simulink model "balanceCar"  (R2023b)
settings: Solver=VariableStepAuto  StartTime=0.0  StopTime=40  RelTol=1e-3
settings Model: Creator=xjtu  LastModifiedBy=xjtu

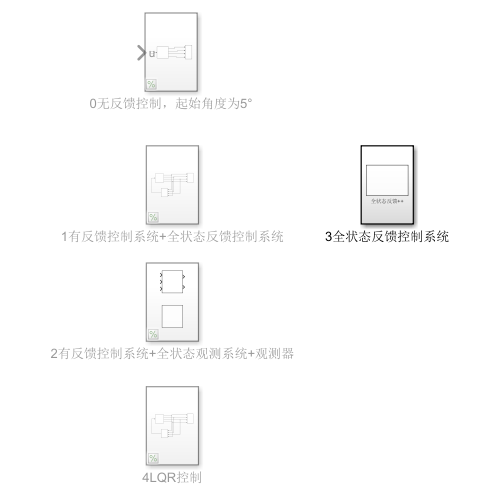
[thumbnail: Simulink's stored preview of the top-level diagram]
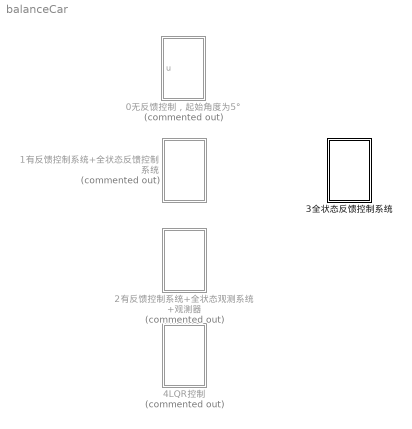
== system balanceCar ==
  0无反馈控制，起始角度为5° : Subsystem  Commented=on
  1有反馈控制系统+全状态反馈控制系统 : Subsystem  Commented=on
  2有反馈控制系统+全状态观测系统+观测器 : Subsystem  Commented=on
  3全状态反馈控制系统 : Subsystem
  4LQR控制 : Subsystem  Commented=on

== system balanceCar/0无反馈控制，起始角度为5° ==
  u : Inport
  Scope : Scope  NumInputPorts=4
  Subsystem : Subsystem
  wires:
  Subsystem/4(dot theta) -> Scope/4
  Subsystem/1(x) -> Scope/1
  u/1 -> Subsystem/1(u)
  Subsystem/2(dot x) -> Scope/2
  Subsystem/3(theta) -> Scope/3

== system balanceCar/1有反馈控制系统+全状态反馈控制系统 ==
  Scope : Scope  NumInputPorts=4
  Subsystem : Subsystem
  Subsystem1 : Subsystem
  wires:
  Subsystem1/3(theta) -> Scope/3, Subsystem/3(theta)
  Subsystem1/4(dot theta) -> Scope/4, Subsystem/4(dot theta)
  Subsystem1/2(dot x) -> Scope/2, Subsystem/2(dot x)
  Subsystem1/1(x) -> Subsystem/1(x), Scope/1
  Subsystem/1(u) -> Subsystem1/1(u)

== system balanceCar/2有反馈控制系统+全状态观测系统+观测器 ==
  全状态观测++ : Subsystem
  可以用来参考学习 : Subsystem

== system balanceCar/3全状态反馈控制系统 ==
  全状态反馈++ : Subsystem

== system balanceCar/4LQR控制 ==
  Scope : Scope  NumInputPorts=4
  Subsystem : Subsystem
  Subsystem1 : Subsystem
  wires:
  Subsystem/1(u) -> Subsystem1/1(u)
  Subsystem1/1(x) -> Scope/1, Subsystem/1(x)
  Subsystem1/2(dot x) -> Subsystem/2(dot x), Scope/2
  Subsystem1/4(dot theta) -> Subsystem/4(dot theta), Scope/4
  Subsystem1/3(theta) -> Subsystem/3(theta), Scope/3

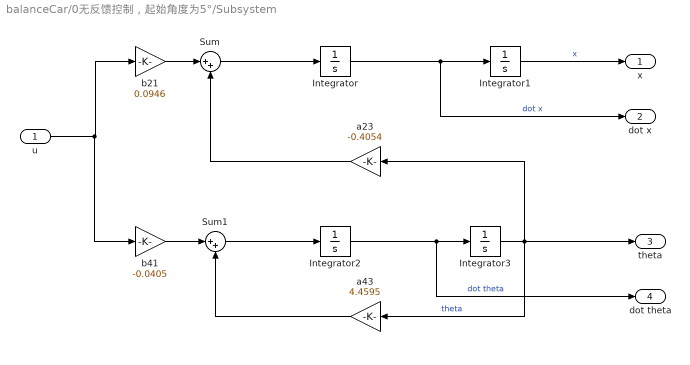
== system balanceCar/0无反馈控制，起始角度为5°/Subsystem ==
  u : Inport
  Integrator : Integrator
  Integrator1 : Integrator
  Integrator2 : Integrator
  Integrator3 : Integrator  InitialCondition=5*pi/180  UpperSaturationLimit=360  LowerSaturationLimit=-360
  Sum : Sum  Inputs=|++
  Sum1 : Sum  Inputs=|++
  a23 : Gain  Gain=-0.4054
  a43 : Gain  Gain=4.4595
  b21 : Gain  Gain=0.0946
  b41 : Gain  Gain=-0.0405
  x : Outport
  dot x : Outport  Port=2
  theta : Outport  Port=3
  dot theta : Outport  Port=4
  wires:
  Integrator2/1 -> dot theta/1, Integrator3/1  "dot theta"
  u/1 -> b41/1, b21/1
  Sum1/1 -> Integrator2/1
  Integrator1/1 -> x/1  "x"
  a23/1 -> Sum/2
  b21/1 -> Sum/1
  Integrator/1 -> dot x/1, Integrator1/1  "dot x"
  Integrator3/1 -> theta/1, a43/1, a23/1  "theta"
  b41/1 -> Sum1/1
  Sum/1 -> Integrator/1
  a43/1 -> Sum1/2

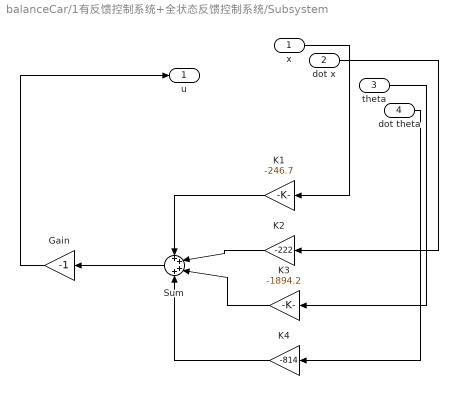
== system balanceCar/1有反馈控制系统+全状态反馈控制系统/Subsystem ==
  x : Inport
  dot x : Inport  Port=2
  theta : Inport  Port=3
  dot theta : Inport  Port=4
  Gain : Gain  Gain=-1
  K1 : Gain  Gain=-246.7
  K2 : Gain  Gain=-222
  K3 : Gain  Gain=-1894.2
  K4 : Gain  Gain=-814
  Sum : Sum  Inputs=++++
  u : Outport
  wires:
  dot theta/1 -> K4/1
  Gain/1 -> u/1
  K2/1 -> Sum/2
  Sum/1 -> Gain/1
  x/1 -> K1/1
  K1/1 -> Sum/1
  K3/1 -> Sum/3
  dot x/1 -> K2/1
  K4/1 -> Sum/4
  theta/1 -> K3/1

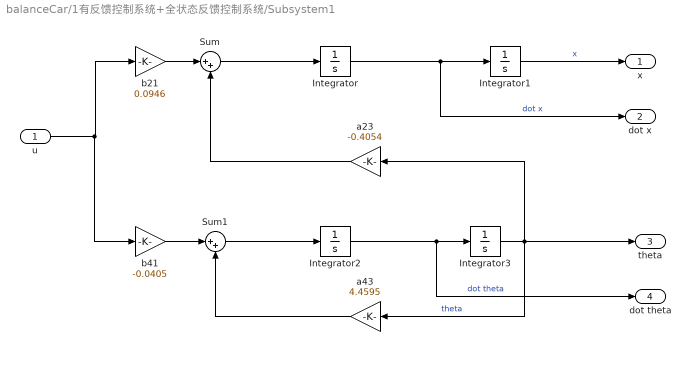
== system balanceCar/1有反馈控制系统+全状态反馈控制系统/Subsystem1 ==
  u : Inport
  Integrator : Integrator
  Integrator1 : Integrator
  Integrator2 : Integrator
  Integrator3 : Integrator  InitialCondition=5*pi/180  UpperSaturationLimit=360  LowerSaturationLimit=-360
  Sum : Sum  Inputs=|++
  Sum1 : Sum  Inputs=|++
  a23 : Gain  Gain=-0.4054
  a43 : Gain  Gain=4.4595
  b21 : Gain  Gain=0.0946
  b41 : Gain  Gain=-0.0405
  x : Outport
  dot x : Outport  Port=2
  theta : Outport  Port=3
  dot theta : Outport  Port=4
  wires:
  a43/1 -> Sum1/2
  Sum/1 -> Integrator/1
  b41/1 -> Sum1/1
  Integrator3/1 -> a23/1, a43/1, theta/1  "theta"
  Integrator/1 -> Integrator1/1, dot x/1  "dot x"
  b21/1 -> Sum/1
  a23/1 -> Sum/2
  Integrator1/1 -> x/1  "x"
  Sum1/1 -> Integrator2/1
  u/1 -> b21/1, b41/1
  Integrator2/1 -> Integrator3/1, dot theta/1  "dot theta"

== system balanceCar/2有反馈控制系统+全状态观测系统+观测器/全状态观测++ ==
  Scope : Scope  NumInputPorts=4
  Subsystem : Subsystem
  Subsystem1 : Subsystem
  Subsystem2 : Subsystem
  位移对比 : Scope  NumInputPorts=2
  角度对比 : Scope  NumInputPorts=2
  角速度对比 : Scope  NumInputPorts=2
  速度对比 : Scope  NumInputPorts=2
  wires:
  Subsystem1/2(dot x) -> Scope/2, 速度对比/1, Subsystem/2(dot x)
  Subsystem1/4(dot theta) -> Scope/4, 角速度对比/1, Subsystem/4(dot theta)
  Subsystem/1(u) -> Subsystem1/1(u)
  Subsystem1/1(x) -> Subsystem2/1(x), 位移对比/1, Scope/1, Subsystem/1(x)
  Subsystem1/3(theta) -> Subsystem2/2(theta), Scope/3, 角度对比/1, Subsystem/3(theta)
  Subsystem2/1(位移x) -> 位移对比/2
  Subsystem2/3(角度 theta) -> 角度对比/2
  Subsystem2/2(速度 dot x) -> 速度对比/2
  Subsystem2/4(角速度 dot theta) -> 角速度对比/2

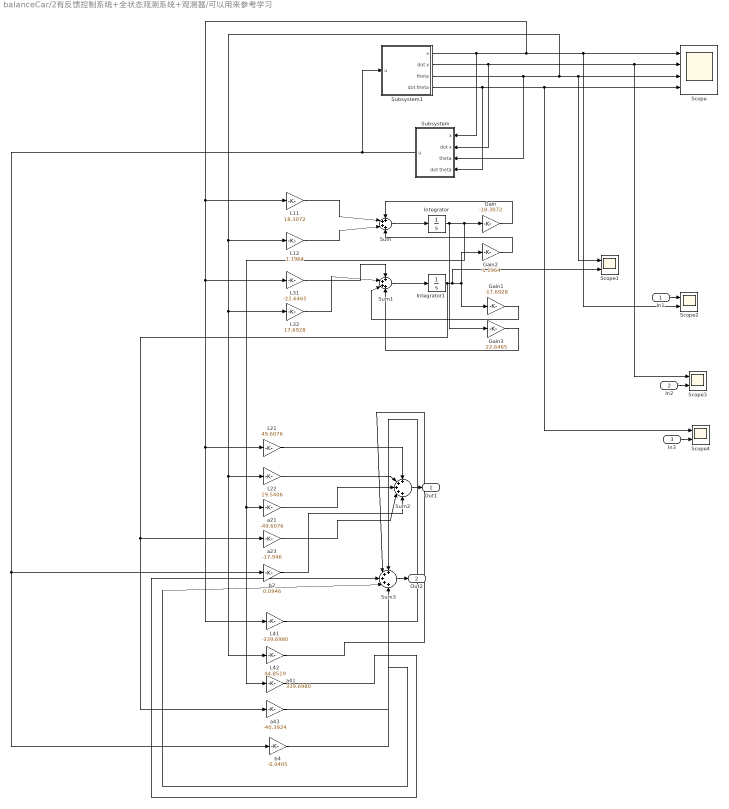
== system balanceCar/2有反馈控制系统+全状态观测系统+观测器/可以用来参考学习 ==
  In1 : Inport
  In2 : Inport  Port=2
  In3 : Inport  Port=3
  Gain : Gain  Gain=-18.3072
  Gain1 : Gain  Gain=-17.6928
  Gain2 : Gain  Gain=-1.1964
  Gain3 : Gain  Gain=22.6465
  Integrator : Integrator
  Integrator1 : Integrator  InitialCondition=pi*5/180
  L11 : Gain  Gain=18.3072
  L12 : Gain  Gain=1.1964
  L21 : Gain  Gain=49.6076
  L22 : Gain  Gain=19.5406
  L31 : Gain  Gain=-22.6465
  L32 : Gain  Gain=17.6928
  L41 : Gain  Gain=-339.6980
  L42 : Gain  Gain=44.8519
  Scope : Scope  NumInputPorts=4
  Scope{1..4} (4 alike) : Scope  NumInputPorts=2
  Subsystem : Subsystem
  Subsystem1 : Subsystem
  Sum : Sum  Inputs=++++
  Sum1 : Sum  Inputs=++++
  Sum2 : Sum  Inputs=+++++
  Sum3 : Sum  Inputs=+++++
  a21 : Gain  Gain=-49.6076
  a23 : Gain  Gain=-17.946
  a41 : Gain  Gain=339.6980
  a43 : Gain  Gain=-40.3924
  b2 : Gain  Gain=0.0946
  b4 : Gain  Gain=-0.0405
  Out1 : Outport
  Out2 : Outport  Port=2
  wires:
  L11/1 -> Sum/2
  L21/1 -> Sum2/1
  Subsystem1/3(theta) -> Subsystem/3(theta), L32/1, L22/1, L42/1, L12/1, Scope1/1, Scope/3
  Gain3/1 -> Sum1/4
  a43/1 -> Sum3/4
  Subsystem1/1(x) -> Subsystem/1(x), L31/1, L21/1, L41/1, L11/1, Scope/1, Scope2/2
  b4/1 -> Sum3/5
  Gain2/1 -> Sum/4
  a41/1 -> Sum3/3
  Integrator1/1 -> Gain2/1, Gain1/1, Scope1/2, a43/1, a23/1
  L42/1 -> Sum3/2
  L22/1 -> Sum2/2
  L32/1 -> Sum1/2
  L31/1 -> Sum1/1
  Subsystem/1(u) -> Subsystem1/1(u), b2/1, b4/1
  Subsystem1/4(dot theta) -> Subsystem/4(dot theta), Scope4/1, Scope/4
  In2/1 -> Scope3/2
  Sum/1 -> Integrator/1
  a23/1 -> Sum2/4
  Subsystem1/2(dot x) -> Subsystem/2(dot x), Scope3/1, Scope/2
  L41/1 -> Sum3/1
  L12/1 -> Sum/3
  Integrator/1 -> Gain3/1, a41/1, a21/1, Gain/1
  Sum1/1 -> Integrator1/1
  b2/1 -> Sum2/5
  a21/1 -> Sum2/3
  Gain/1 -> Sum/1
  Gain1/1 -> Sum1/3
  Sum2/1 -> Out1/1
  Sum3/1 -> Out2/1
  In1/1 -> Scope2/1
  In3/1 -> Scope4/2

== system balanceCar/3全状态反馈控制系统/全状态反馈++ ==
  Scope : Scope  NumInputPorts=4
  Subsystem : Subsystem
  Subsystem1 : Subsystem
  Subsystem2 : Subsystem
  位移对比 : Scope  NumInputPorts=2
  角度对比 : Scope  NumInputPorts=2
  角速度对比 : Scope  NumInputPorts=2
  速度对比 : Scope  NumInputPorts=2
  wires:
  Subsystem1/2(dot x) -> 速度对比/1, Scope/2, Subsystem/2(dot x)
  Subsystem2/4(角速度 dot theta) -> 角速度对比/2
  Subsystem1/3(theta) -> Subsystem/3(theta), 角度对比/1, Scope/3, Subsystem2/2(theta)
  Subsystem1/1(x) -> Subsystem/1(x), Scope/1, 位移对比/1, Subsystem2/1(x)
  Subsystem/1(u) -> Subsystem1/1(u)
  Subsystem2/1(位移x) -> 位移对比/2
  Subsystem2/3(角度 theta) -> 角度对比/2
  Subsystem2/2(速度 dot x) -> 速度对比/2
  Subsystem1/4(dot theta) -> Subsystem/4(dot theta), 角速度对比/1, Scope/4

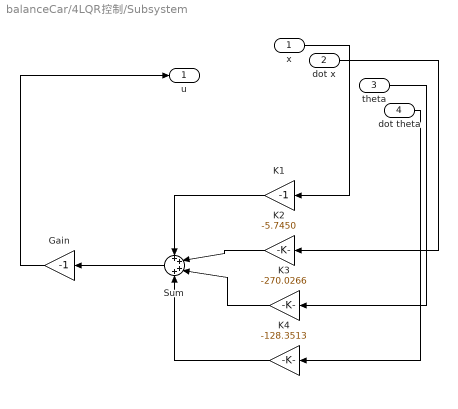
== system balanceCar/4LQR控制/Subsystem ==
  x : Inport
  dot x : Inport  Port=2
  theta : Inport  Port=3
  dot theta : Inport  Port=4
  Gain : Gain  Gain=-1
  K1 : Gain  Gain=-1
  K2 : Gain  Gain=-5.7450
  K3 : Gain  Gain=-270.0266
  K4 : Gain  Gain=-128.3513
  Sum : Sum  Inputs=++++
  u : Outport
  wires:
  theta/1 -> K3/1
  K4/1 -> Sum/4
  dot x/1 -> K2/1
  K3/1 -> Sum/3
  K1/1 -> Sum/1
  x/1 -> K1/1
  Sum/1 -> Gain/1
  K2/1 -> Sum/2
  Gain/1 -> u/1
  dot theta/1 -> K4/1

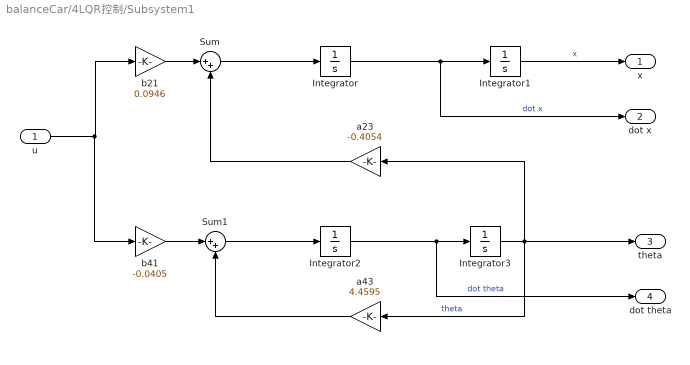
== system balanceCar/4LQR控制/Subsystem1 ==
  u : Inport
  Integrator : Integrator
  Integrator1 : Integrator
  Integrator2 : Integrator
  Integrator3 : Integrator  InitialCondition=5*pi/180  UpperSaturationLimit=360  LowerSaturationLimit=-360
  Sum : Sum  Inputs=|++
  Sum1 : Sum  Inputs=|++
  a23 : Gain  Gain=-0.4054
  a43 : Gain  Gain=4.4595
  b21 : Gain  Gain=0.0946
  b41 : Gain  Gain=-0.0405
  x : Outport
  dot x : Outport  Port=2
  theta : Outport  Port=3
  dot theta : Outport  Port=4
  wires:
  Integrator2/1 -> dot theta/1, Integrator3/1  "dot theta"
  u/1 -> b41/1, b21/1
  Sum1/1 -> Integrator2/1
  Integrator1/1 -> x/1  "x"
  a23/1 -> Sum/2
  b21/1 -> Sum/1
  Integrator/1 -> dot x/1, Integrator1/1  "dot x"
  Integrator3/1 -> theta/1, a43/1, a23/1  "theta"
  b41/1 -> Sum1/1
  Sum/1 -> Integrator/1
  a43/1 -> Sum1/2

== system balanceCar/2有反馈控制系统+全状态观测系统+观测器/全状态观测++/Subsystem ==
  x : Inport
  dot x : Inport  Port=2
  theta : Inport  Port=3
  dot theta : Inport  Port=4
  Gain : Gain  Gain=-1
  K1 : Gain  Gain=-246.7
  K2 : Gain  Gain=-222
  K3 : Gain  Gain=-1894.2
  K4 : Gain  Gain=-814
  Sum : Sum  Inputs=++++
  u : Outport
  wires:
  dot theta/1 -> K4/1
  Gain/1 -> u/1
  K2/1 -> Sum/2
  Sum/1 -> Gain/1
  x/1 -> K1/1
  K1/1 -> Sum/1
  K3/1 -> Sum/3
  dot x/1 -> K2/1
  K4/1 -> Sum/4
  theta/1 -> K3/1

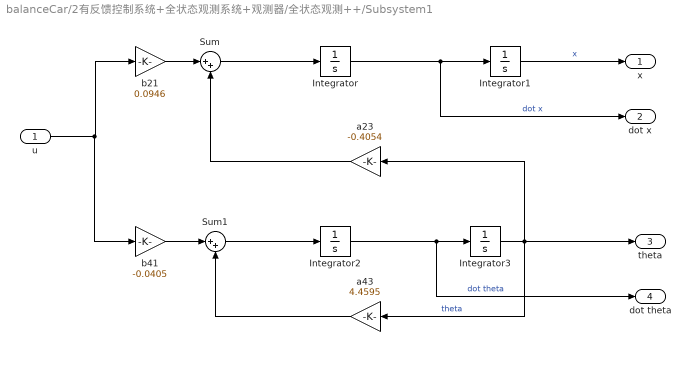
== system balanceCar/2有反馈控制系统+全状态观测系统+观测器/全状态观测++/Subsystem1 ==
  u : Inport
  Integrator : Integrator
  Integrator1 : Integrator
  Integrator2 : Integrator
  Integrator3 : Integrator  InitialCondition=5*pi/180  UpperSaturationLimit=360  LowerSaturationLimit=-360
  Sum : Sum  Inputs=|++
  Sum1 : Sum  Inputs=|++
  a23 : Gain  Gain=-0.4054
  a43 : Gain  Gain=4.4595
  b21 : Gain  Gain=0.0946
  b41 : Gain  Gain=-0.0405
  x : Outport
  dot x : Outport  Port=2
  theta : Outport  Port=3
  dot theta : Outport  Port=4
  wires:
  a43/1 -> Sum1/2
  Sum/1 -> Integrator/1
  b41/1 -> Sum1/1
  Integrator3/1 -> a23/1, a43/1, theta/1  "theta"
  Integrator/1 -> Integrator1/1, dot x/1  "dot x"
  b21/1 -> Sum/1
  a23/1 -> Sum/2
  Integrator1/1 -> x/1  "x"
  Sum1/1 -> Integrator2/1
  u/1 -> b21/1, b41/1
  Integrator2/1 -> Integrator3/1, dot theta/1  "dot theta"

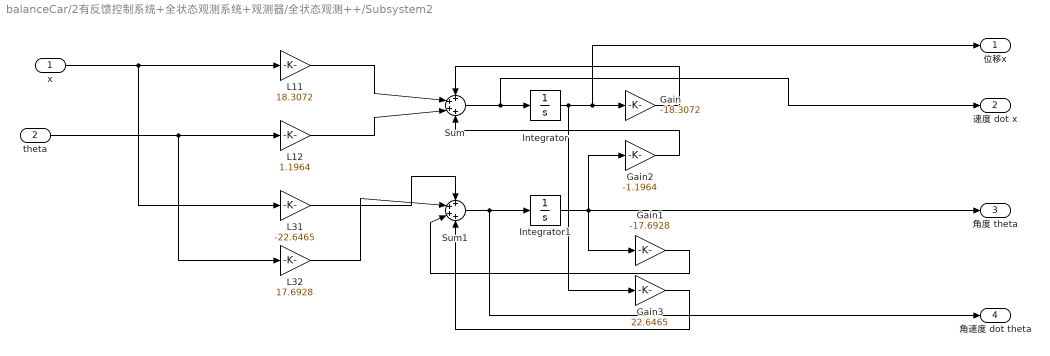
== system balanceCar/2有反馈控制系统+全状态观测系统+观测器/全状态观测++/Subsystem2 ==
  x : Inport
  theta : Inport  Port=2
  Gain : Gain  Gain=-18.3072
  Gain1 : Gain  Gain=-17.6928
  Gain2 : Gain  Gain=-1.1964
  Gain3 : Gain  Gain=22.6465
  Integrator : Integrator
  Integrator1 : Integrator
  L11 : Gain  Gain=18.3072
  L12 : Gain  Gain=1.1964
  L31 : Gain  Gain=-22.6465
  L32 : Gain  Gain=17.6928
  Sum : Sum  Inputs=++++
  Sum1 : Sum  Inputs=++++
  位移x : Outport
  速度 dot x : Outport  Port=2
  角度 theta : Outport  Port=3
  角速度 dot theta : Outport  Port=4
  wires:
  L31/1 -> Sum1/1
  Sum/1 -> 速度 dot x/1, Integrator/1
  Gain/1 -> Sum/1
  Sum1/1 -> 角速度 dot theta/1, Integrator1/1
  Integrator1/1 -> 角度 theta/1, Gain1/1, Gain2/1
  L11/1 -> Sum/2
  theta/1 -> L12/1, L32/1
  Integrator/1 -> 位移x/1, Gain/1, Gain3/1
  Gain1/1 -> Sum1/3
  L32/1 -> Sum1/2
  Gain2/1 -> Sum/4
  x/1 -> L11/1, L31/1
  Gain3/1 -> Sum1/4
  L12/1 -> Sum/3

== system balanceCar/2有反馈控制系统+全状态观测系统+观测器/可以用来参考学习/Subsystem ==
  x : Inport
  dot x : Inport  Port=2
  theta : Inport  Port=3
  dot theta : Inport  Port=4
  Gain : Gain  Gain=-1
  K1 : Gain  Gain=-246.7
  K2 : Gain  Gain=-222
  K3 : Gain  Gain=-1894.2
  K4 : Gain  Gain=-814
  Sum : Sum  Inputs=++++
  u : Outport
  wires:
  theta/1 -> K3/1
  K4/1 -> Sum/4
  dot x/1 -> K2/1
  K3/1 -> Sum/3
  K1/1 -> Sum/1
  x/1 -> K1/1
  Sum/1 -> Gain/1
  K2/1 -> Sum/2
  Gain/1 -> u/1
  dot theta/1 -> K4/1

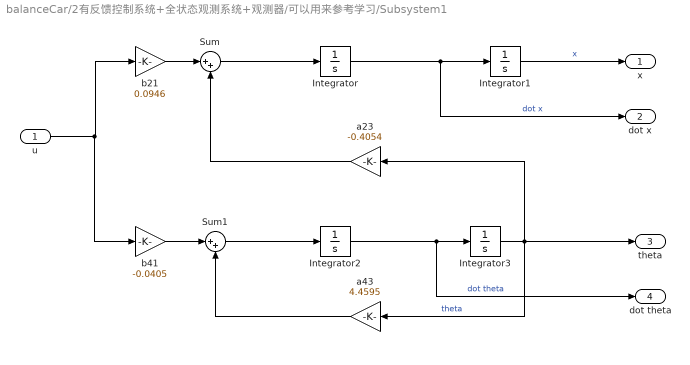
== system balanceCar/2有反馈控制系统+全状态观测系统+观测器/可以用来参考学习/Subsystem1 ==
  u : Inport
  Integrator : Integrator
  Integrator1 : Integrator
  Integrator2 : Integrator
  Integrator3 : Integrator  InitialCondition=5*pi/180  UpperSaturationLimit=360  LowerSaturationLimit=-360
  Sum : Sum  Inputs=|++
  Sum1 : Sum  Inputs=|++
  a23 : Gain  Gain=-0.4054
  a43 : Gain  Gain=4.4595
  b21 : Gain  Gain=0.0946
  b41 : Gain  Gain=-0.0405
  x : Outport
  dot x : Outport  Port=2
  theta : Outport  Port=3
  dot theta : Outport  Port=4
  wires:
  Integrator2/1 -> dot theta/1, Integrator3/1  "dot theta"
  u/1 -> b41/1, b21/1
  Sum1/1 -> Integrator2/1
  Integrator1/1 -> x/1  "x"
  a23/1 -> Sum/2
  b21/1 -> Sum/1
  Integrator/1 -> dot x/1, Integrator1/1  "dot x"
  Integrator3/1 -> theta/1, a43/1, a23/1  "theta"
  b41/1 -> Sum1/1
  Sum/1 -> Integrator/1
  a43/1 -> Sum1/2

== system balanceCar/3全状态反馈控制系统/全状态反馈++/Subsystem ==
  x : Inport
  dot x : Inport  Port=2
  theta : Inport  Port=3
  dot theta : Inport  Port=4
  Gain : Gain  Gain=-1
  K1 : Gain  Gain=-246.7
  K2 : Gain  Gain=-222
  K3 : Gain  Gain=-1894.2
  K4 : Gain  Gain=-814
  Sum : Sum  Inputs=++++
  u : Outport
  wires:
  theta/1 -> K3/1
  K4/1 -> Sum/4
  dot x/1 -> K2/1
  K3/1 -> Sum/3
  K1/1 -> Sum/1
  x/1 -> K1/1
  Sum/1 -> Gain/1
  K2/1 -> Sum/2
  Gain/1 -> u/1
  dot theta/1 -> K4/1

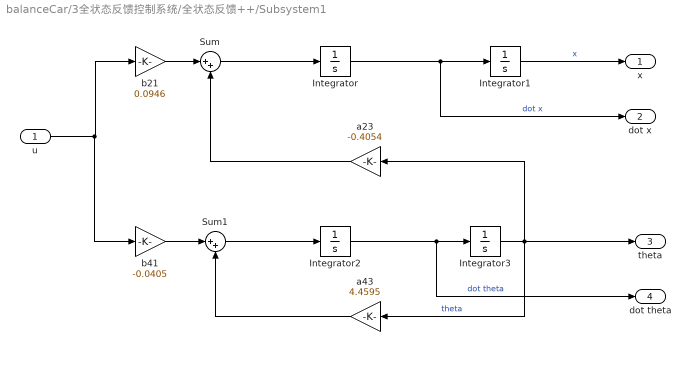
== system balanceCar/3全状态反馈控制系统/全状态反馈++/Subsystem1 ==
  u : Inport
  Integrator : Integrator
  Integrator1 : Integrator
  Integrator2 : Integrator
  Integrator3 : Integrator  InitialCondition=5*pi/180  UpperSaturationLimit=360  LowerSaturationLimit=-360
  Sum : Sum  Inputs=|++
  Sum1 : Sum  Inputs=|++
  a23 : Gain  Gain=-0.4054
  a43 : Gain  Gain=4.4595
  b21 : Gain  Gain=0.0946
  b41 : Gain  Gain=-0.0405
  x : Outport
  dot x : Outport  Port=2
  theta : Outport  Port=3
  dot theta : Outport  Port=4
  wires:
  Integrator2/1 -> dot theta/1, Integrator3/1  "dot theta"
  u/1 -> b41/1, b21/1
  Sum1/1 -> Integrator2/1
  Integrator1/1 -> x/1  "x"
  a23/1 -> Sum/2
  b21/1 -> Sum/1
  Integrator/1 -> dot x/1, Integrator1/1  "dot x"
  Integrator3/1 -> theta/1, a43/1, a23/1  "theta"
  b41/1 -> Sum1/1
  Sum/1 -> Integrator/1
  a43/1 -> Sum1/2

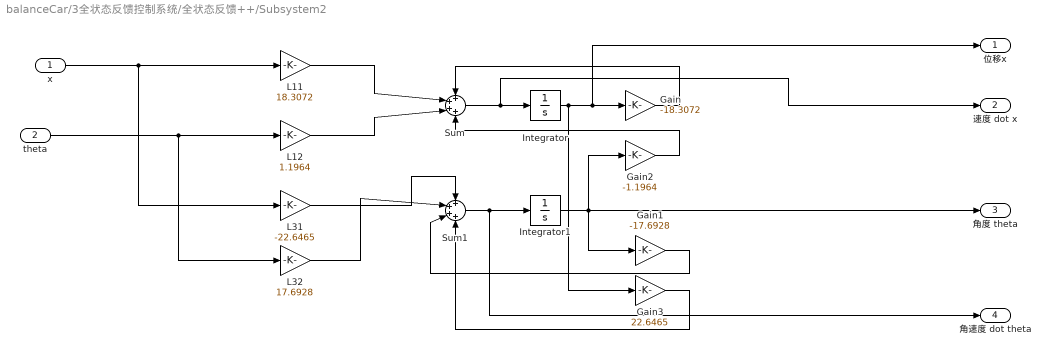
== system balanceCar/3全状态反馈控制系统/全状态反馈++/Subsystem2 ==
  x : Inport
  theta : Inport  Port=2
  Gain : Gain  Gain=-18.3072
  Gain1 : Gain  Gain=-17.6928
  Gain2 : Gain  Gain=-1.1964
  Gain3 : Gain  Gain=22.6465
  Integrator : Integrator
  Integrator1 : Integrator
  L11 : Gain  Gain=18.3072
  L12 : Gain  Gain=1.1964
  L31 : Gain  Gain=-22.6465
  L32 : Gain  Gain=17.6928
  Sum : Sum  Inputs=++++
  Sum1 : Sum  Inputs=++++
  位移x : Outport
  速度 dot x : Outport  Port=2
  角度 theta : Outport  Port=3
  角速度 dot theta : Outport  Port=4
  wires:
  L12/1 -> Sum/3
  Gain3/1 -> Sum1/4
  x/1 -> L31/1, L11/1
  Gain2/1 -> Sum/4
  L32/1 -> Sum1/2
  Gain1/1 -> Sum1/3
  Integrator/1 -> Gain3/1, Gain/1, 位移x/1
  theta/1 -> L32/1, L12/1
  L11/1 -> Sum/2
  Integrator1/1 -> Gain2/1, Gain1/1, 角度 theta/1
  Sum1/1 -> Integrator1/1, 角速度 dot theta/1
  Gain/1 -> Sum/1
  Sum/1 -> Integrator/1, 速度 dot x/1
  L31/1 -> Sum1/1
